simulink model "Super13"  (Simulink 6.0)
settings: Solver=ode45  StartTime=0.0  StopTime=10.0  RelTol=1e-3
settings Model: Creator=scaife  LastModifiedBy=scaife  ExtModeAutoUpdateStatusClock=off
settings DataIOCC: SignalLoggingName=sigsOut
settings DebuggingCC: SolverPrmCheckMsg=none
settings HardwareCC: TargetUnknown=on
settings STFCustomTargetCC: TargetFcnLib=ansi_tfl_tmw.mat  GenFloatMathFcnCalls=ANSI_C  ModelReferenceCompliant=off  SystemTargetFile=grt.tlc

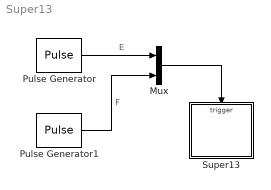
== system Super13 ==
  Mux : Mux  Inputs=2
  Pulse Generator : DiscretePulseGenerator
  Pulse Generator1 : DiscretePulseGenerator  Period=4  PulseWidth=2
  Super13 : Stateflow chart
  wires:
  Mux/1 -> Super13/Trigger
  Pulse Generator/1 -> Mux/1  "E"
  Pulse Generator1/1 -> Mux/2  "F"

== stateflow chart Super13 ==
  state A
    state A1
    (default) -> A1
  state C
  state B
  C -> A1 : E
  (default) -> C
  A1 -> C : F
  A -> B : E
  events: E input EITHER_EDGE_EVENT; F input EITHER_EDGE_EVENT
